simulink library "ITKLib"  (R2022b)
settings: Solver=FixedStepDiscrete  StartTime=0.0  StopTime=10.0  FixedStep=0.01  RelTol=1e-3  EnableMultiTasking=on
values from neighbouring files (symbols this model uses):
  Glb_WhlRollgRd_SC = single(0.36)    [init_Global.m]
undefined symbols (not defined in the file or in its folder): docblock, SlDemoSign, SlDemoSign_Positive_SC, TaskTime_100ms_SC, TaskTime_10ms_SC, VehRefSpd_vMaxRefSpd_C
libraries: simulink x51, $bdroot x45, ITKLib_V14 x1
(part 1 of 10)
settings Model: Creator=MaoChongchong  LastModifiedBy=shuli1
settings SolverCC: AlgebraicLoopSolver=TrustRegion
settings DataIOCC: LimitDataPoints=on  SaveOutput=off  SaveTime=off  ReturnWorkspaceOutputs=off
settings OptimizationCC: DefaultParameterBehavior=Inlined  LifeSpan=1  EfficientTunableParamExpr=on
settings DebuggingCC: UnconnectedInputMsg=warning  UnconnectedOutputMsg=warning  UnconnectedLineMsg=warning  AllowSymbolicDim=off  SFUnexpectedBacktrackingDiag=warning  SFNoUnconditionalDefaultTransitionDiag=warning  SFExecutionAtInitializationDiag=none  SFMachineParentedDataDiag=warning  ArithmeticOperatorsInVariantConditions=warning
settings ModelReferenceCC: EnableRefExpFcnMdlSchedulingChecks=on  PropagateSignalLabelsOutOfModel=off
settings SFSimCC: SimUseLocalCustomCode=off  MATLABDynamicMemAlloc=off  CustomCodeUndefinedFunction=UseInterfaceOnly
settings RTWCC: Description=Embedded Coder  SystemTargetFile=ert.tlc  TemplateMakefile=ert_default_tmf  RTWUseLocalCustomCode=off  DLArmComputeVersion=19.05
settings CodeAppCC: IgnoreCustomStorageClasses=off  StateflowObjectComments=on
settings ERTTargetCC: MultiwordLength=2048  GenerateSampleERTMain=on  InlinedParameterPlacement=NonHierarchical  ERTCustomFileTemplate=example_file_process.tlc  ConvertIfToSwitch=off  SuppressUnreachableDefaultCases=off
settings ConfigComp: CovMetricSettings=dw  CovSaveCumulativeToWorkspaceVar=on  CovSaveSingleToWorkspaceVar=on  CovExternalEMLEnable=off

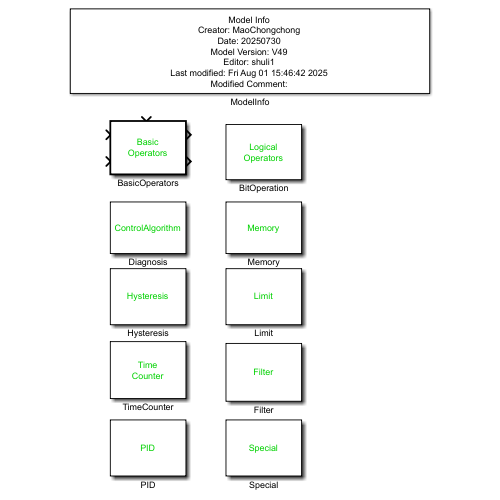
[thumbnail: Simulink's stored preview of the top-level diagram]
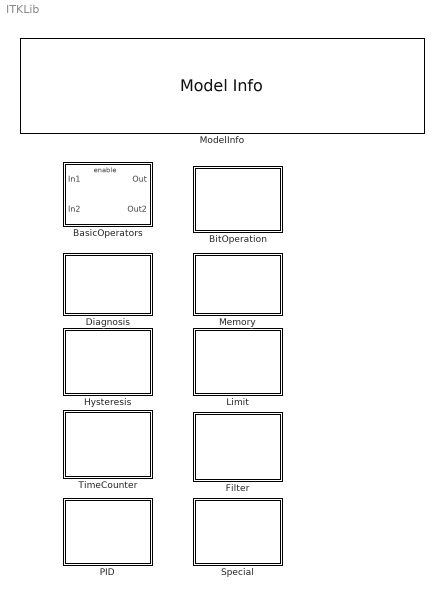
== system ITKLib ==
  BasicOperators : Subsystem
      mask Display:
      | color('green')
      | fprintf('Basic\nOperators')
  BitOperation : Subsystem
      mask Display:
      | color('green')
      | fprintf('Logical\nOperators')
  Diagnosis : Subsystem
      mask Display:
      | color('green')
      | fprintf('ControlAlgorithm')
  Filter : Subsystem
      mask Display:
      | color('green')
      | fprintf('Filter')
  Hysteresis : Subsystem
      mask Display:
      | color('green')
      | fprintf('Hysteresis')
  Limit : Subsystem
      mask Display:
      | color('green')
      | fprintf('Limit')
  Memory : Subsystem
      mask Display:
      | color('green')
      | fprintf('Memory')
  ModelInfo : simulink/Model-Wide Utilities/Model Info  Frame=on  DisplayStringWithTags=|  HorizontalTextAlignment=Center  LeftAlignmentValue=0.5
      | Model Info
      | Creator: MaoChongchong
      | Date: 20250730
      | Model Version: V49
      | Editor: %<LastModifiedBy>
      | Last modified: %<ModifiedDate>
      | Modified Comment:
  PID : Subsystem
      mask Display:
      | color('green')
      | fprintf('PID')
  Special : Subsystem  Description=Refer Detailed Function Description for detailed information.
      mask Display:
      | color('green')
      | fprintf('Special')
  TimeCounter : Subsystem
      mask Display:
      | color('green')
      | fprintf('Time\nCounter')

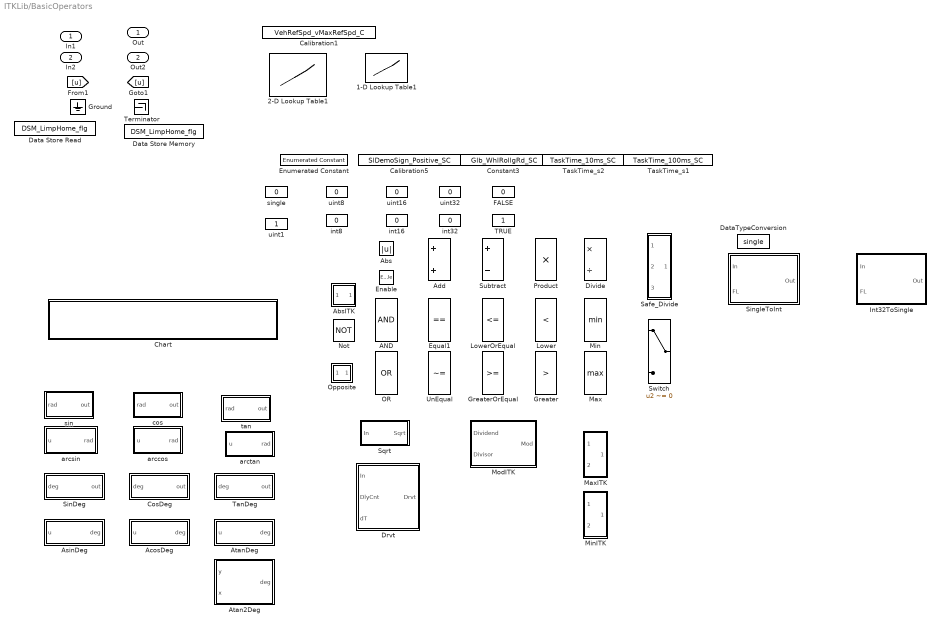
== system ITKLib/BasicOperators ==
  In1 : Inport
  In2 : Inport  Port=2
  Enable : EnablePort
  1-D Lookup Table1 : Lookup_n-D  NumberOfTableDimensions=1  BreakpointsForDimension1=[-5:5]  BreakpointsForDimension1DataTypeStr=Inherit: Inherit from 'Breakpoint data'  Table=tanh([-5:5])  TableDataTypeStr=Inherit: Inherit from 'Table data'  ExtrapMethod=Clip  UseLastTableValue=on  InternalRulePriority=Speed  OutDataTypeStr=Inherit: Inherit from 'Table data'  RndMeth=Simplest
      settings: AttributesFormatString=|
      | input = %<BreakpointsForDimension1>
      | output = %<Table>
      | extrapolation-use end values: %<UseLastTableValue>
  2-D Lookup Table1 : Lookup_n-D  BreakpointsForDimension1=[1:3]  BreakpointsForDimension2=[1:3]  BreakpointsForDimension1DataTypeStr=Inherit: Inherit from 'Breakpoint data'  BreakpointsForDimension2DataTypeStr=Inherit: Inherit from 'Breakpoint data'  TableDataTypeStr=Inherit: Inherit from 'Table data'  ExtrapMethod=Clip  UseLastTableValue=on  InternalRulePriority=Speed  OutDataTypeStr=Inherit: Inherit from 'Table data'  RndMeth=Simplest  InputSameDT=off
      settings: InputPortMap=u0,u1
      settings: AttributesFormatString=|
      | row = %<BreakpointsForDimension1>
      | column = %<BreakpointsForDimension2>
      | output = %<Table>
      | extrapolation-use end values: %<UseLastTableValue>
  AND : Logic  OutDataTypeStr=boolean
  Abs : Abs  SaturateOnIntegerOverflow=off  OutDataTypeStr=Inherit: Inherit via internal rule
  AbsITK : Subsystem  mask(AbsITK){}
      mask help: This block returns the absolute value of input
      mask Display:
      | color('blue')
      | disp('\fontsize{12}Abs', 'texmode', 'on')
      | color('green');
      | text(1,0,'ITK','horizontalAlignment','right','verticalAlignment','bottom');
  AcosDeg : Subsystem  mask(Acos){}
      mask help:
      | This block returns the sin of an angle
      | Result = acos(value)
      | Input:
      |             u: input value, the maximum value is 1, the minimum value is -1;
      | Output:
      |             out: angle, unit: deg, the maximum value is 180 deg, the minimum value is 0 deg;
      mask Display:
      | color('blue')
      | disp('\fontsize{10}acos', 'texmode', 'on')
      | color('green');
      | text(1,0,'ITK','horizontalAlignment','right','verticalAlignment','bottom');
  Add : Sum  InputSameDT=on  SaturateOnIntegerOverflow=on
  AsinDeg : Subsystem  mask(AsinDeg){}
      mask help:
      | This block returns the sin of an angle
      | Result = asin(value)
      | Input:
      |             u: input value, the maximum value is 1, the minimum value is -1;
      | Output:
      |             out: angle, unit: deg, the maximum value is 90 deg, the minimum value is -90 deg;
      mask Display:
      | color('blue')
      | disp('\fontsize{10}asin', 'texmode', 'on')
      | color('green');
      | text(1,0,'ITK','horizontalAlignment','right','verticalAlignment','bottom');
  Atan2Deg : Subsystem  mask(Atan2Deg){}
      mask help:
      | This block returns the sin of an angle
      | Result = atan2(value)
      | Input:
      |             u: input value, the maximum value is 5729, the minimum value is -5729;
      | Output:
      |             out: angle, unit: deg, the maximum value is 179.99 deg, the minimum value is -179.99 deg, does not include from -89.99 deg to -90 deg and from 89.99 deg to 90 deg;
      mask Display:
      | color('blue')
      | disp('\fontsize{10}atan2', 'texmode', 'on')
      | color('green');
      | text(1,0,'ITK','horizontalAlignment','right','verticalAlignment','bottom');
  AtanDeg : Subsystem  mask(Atan){}
      mask help:
      | This block returns the sin of an angle
      | Result = atan(value)
      | Input:
      |             u: input value, the maximum value is 5729, the minimum value is -5729;
      | Output:
      |             out: angle, unit: deg, the maximum value is 89.99 deg, the minimum value is -89.99 deg;
      mask Display:
      | color('blue')
      | disp('\fontsize{10}atan', 'texmode', 'on')
      | color('green');
      | text(1,0,'ITK','horizontalAlignment','right','verticalAlignment','bottom');
  Calibration1 : Constant  Description=[300]  Value=VehRefSpd_vMaxRefSpd_C  SampleTime=-1
      settings: AttributesFormatString=%<Description>
  Calibration5 : Constant  Description=[0]  Value=SlDemoSign_Positive_SC  SampleTime=-1
      settings: AttributesFormatString=%<Description>
  Chart : Stateflow chart  TreatAsAtomicUnit=on
  Constant3 : Constant  Description=[0.36]  Value=Glb_WhlRollgRd_SC  SampleTime=-1
      settings: AttributesFormatString=%<Description>
  CosDeg : Subsystem  mask(CosDeg){}
      mask help:
      | This block returns the sin of an angle
      | Result = cos(value)
      | Input:
      |             deg: input angle, unit: deg, the minimum value is -inf, the maximum value is inf;
      | Output:
      | out: the minimum value is -1, the maximum value is 1;
      mask Display:
      | color('blue')
      | disp('\fontsize{10}cos(deg)', 'texmode', 'on')
      | color('green');
      | text(1,0,'ITK','horizontalAlignment','right','verticalAlignment','bottom');
  Data Store Memory : DataStoreMemory  DataStoreName=DSM_LimpHome_flg  ReadBeforeWriteMsg=warning  WriteAfterWriteMsg=warning  WriteAfterReadMsg=warning  ShowAdditionalParam=off  OutDataTypeStr=boolean
  Data Store Read : DataStoreRead  DataStoreName=DSM_LimpHome_flg  DataStoreElements=DSM_LimpHome_flg  IndexOptions=Index vector (dialog)  Indices=1  OutputSizes=1
  DataTypeConversion : DataTypeConversion  OutDataTypeStr=single  RndMeth=Nearest  SaturateOnIntegerOverflow=off
  Divide : Product  Inputs=*/  InputSameDT=on  SaturateOnIntegerOverflow=on
  Drvt : Subsystem  mask(Drvt){}
      mask help:
      | This block returns the derivativee value of input signal.
      |
      | Input signals:
      |             In: input signal, single data type;
      |             DlyCnt: delay counter value, uint data type;
      |             dT: sample time, single data type, unit is s;
      | Output:
      |             Drvt: derivativee value of In, single data type;
      settings: MinAlgLoopOccurrences=on
      mask Display:
      | color('blue')
      | % disp('\fontsize{10}Drvt', 'texmode', 'on')
      | color('green');
      | % image('SqrtImage.jpg', 'center');
      | image('DrvtImage.jpg', [0.36, 0.3, 0.42, 0.5]);
      | text(1,0,'ITK','horizontalAlignment','right','verticalAlignment','bottom');
  Enumerated Constant : simulink/Sources/Enumerated Constant  OutDataTypeStr=Enum: SlDemoSign  Value=SlDemoSign.Positive  SampleTime=-1
  Equal1 : RelationalOperator  Operator===  OutDataTypeStr=boolean
  FALSE : Constant  Description=FALSE  Value=0  OutDataTypeStr=boolean  SampleTime=-1
      settings: AttributesFormatString=%<Description>
  Greater : RelationalOperator  Operator=>  OutDataTypeStr=boolean
  GreaterOrEqual : RelationalOperator  OutDataTypeStr=boolean
  Ground : Ground
  Int32ToSingle : Subsystem  mask(Int32ToSingle){}
      mask help:
      | Convert int32 number to single number using binary point scaling with specified fraction length (FL).
      | Equivalent to fixdt(1,32,FL) from Fix-point Designer toolbox
      | Input:
      |             In: input signal, int32 data type;
      |             FL: specified fraction length, single data type, ＞0；
      | Output:
      |             Out: output signal, single data type;
      mask Display:
      | color('blue')
      | disp('\fontsize{10}Int32ToSingle', 'texmode', 'on')
      | color('green');
      | % image('SqrtImage.jpg', 'center');
      | % image('SqrtImage.jpg', [0.25, 0.2, 0.4, 0.6]);
      | text(1,0,'ITK','horizontalAlignment','right','verticalAlignment','bottom');
  Lower : RelationalOperator  Operator=<  OutDataTypeStr=boolean
  LowerOrEqual : RelationalOperator  Operator=<=  OutDataTypeStr=boolean
  Max : MinMax  Function=max  Inputs=2  InputSameDT=on  SaturateOnIntegerOverflow=on
  MaxITK : Subsystem  mask(MaxITK){}
      mask help: This block returns the maximal value of input
      mask Display:
      | color('blue')
      | disp('\fontsize{12}Max', 'texmode', 'on')
      | color('green');
      | text(1,0,'ITK','horizontalAlignment','right','verticalAlignment','bottom');
  Min : MinMax  Inputs=2  InputSameDT=on  SaturateOnIntegerOverflow=on
  MinITK : Subsystem  mask(MinITK){}
      mask help: This block returns the minimum value of input
      mask Display:
      | color('blue')
      | disp('\fontsize{12}Min', 'texmode', 'on')
      | color('green');
      | text(1,0,'ITK','horizontalAlignment','right','verticalAlignment','bottom');
  ModITK : Subsystem  mask(ModITK){}
      mask help:
      | This block returns the mod of Dividend/Divisor.
      | Mod = Dividend - fix(Dividend/Divisor)*Divisor
      | Input:
      |             Dividend: ＞0
      |             Divisor: ;＞0
      | Output:
      |             Mod: ;
      mask Display:
      | color('blue')
      | disp('\fontsize{12}Mod', 'texmode', 'on')
      | color('green');
      | % image('SqrtImage.jpg', 'center');
      | % image('SqrtImage.jpg', [0.25, 0.2, 0.4, 0.6]);
      | text(1,0,'ITK','horizontalAlignment','right','verticalAlignment','bottom');
  Not : Logic  Operator=NOT  AllPortsSameDT=off  OutDataTypeStr=boolean
  OR : Logic  Operator=OR  OutDataTypeStr=boolean
  Opposite : Subsystem  RTWFcnName=Minus  RTWFileName=MCC_Mdl_Lib  mask(Opposite){}
      mask help:
      | output = - input;
      | Simulink Custom Model Library, created by MCC.
      settings: RTWFcnNameOpts=User specified  RTWFileNameOpts=User specified
      mask Display:
      | color('blue')
      | fprintf('-ln  ')
      | color('green');
      | % text(1,0,'SEN','horizontalAlignment','right','verticalAlignment','bottom');
  Product : Product  InputSameDT=on  SaturateOnIntegerOverflow=on
  Safe_Divide : Subsystem  RTWFcnName=Safe_Divide  RTWFileName=BoschITK_Mdl_Lib  mask(Safe_Divide){}
      mask help:
      | Safe Divide, prevents division by zero.
      |
      | if abs(denominator) > abs(eps) then
      |     output = numerator / denominator
      | elseif  denominator ≥ 0
      |     output = numerator / abs(eps)
      | else
      |     output = numerator / (-abs(eps))
      |
      |
      | Warning!
      | Use this block only when there is a risk for division by zero.
      |
      | Simulink Custom Model Library, created by MCC.
      settings: RTWFcnNameOpts=User specified  RTWFileNameOpts=User specified
      mask Display:
      | port_label('input', 1, 'x')
      | port_label('input', 2, '÷')
      | port_label('input', 3, 'eps')
  SinDeg : Subsystem  mask(SinDeg){}
      mask help:
      | This block returns the sin of an angle
      | Result = sin(value)
      | Input:
      |             deg: input angle, unit: deg, the minimum value is -inf, the maximum value is inf;
      | Output:
      | out: the minimum value is -1, the maximum value is 1;
      mask Display:
      | color('blue')
      | disp('\fontsize{10}sin(deg)', 'texmode', 'on')
      | color('green');
      | text(1,0,'ITK','horizontalAlignment','right','verticalAlignment','bottom');
  SingleToInt : Subsystem  mask(SingleToInt32){}
      mask help:
      | Convert single number to int32 number using binary point scaling with specified fraction length (FL).
      | Equivalent to fixdt(1,32,FL) from Fix-point Designer toolbox.
      | Input:
      |             In: input signal, single data type;
      |             FL: specified fraction length, single data type, ＞0；
      | Output:
      |             Out: output signal, int32 data type;
      mask Display:
      | color('blue')
      | disp('\fontsize{10}SingleToInt32', 'texmode', 'on')
      | color('green');
      | % image('SqrtImage.jpg', 'center');
      | % image('SqrtImage.jpg', [0.25, 0.2, 0.4, 0.6]);
      | text(1,0,'ITK','horizontalAlignment','right','verticalAlignment','bottom');
  Sqrt : Subsystem  mask(Sqrt){}
      mask help:
      | This block returns the square root value of input signal, according to Newton's iterative method.
      | Sqrt = sqrt(In)
      | Input:
      |             In: input signal, ≥0;
      | Output:
      |             Sqrt: the square root of In, ≥0;
      |  If 0≤ In ≤ 1e13, the output signal Sqrt is right, it has no error;
      |  If  In ＞ 1e13, the output signal Sqrt is not right, it will generate big error;
      mask Display:
      | color('blue')
      | disp('\fontsize{10}Sqrt', 'texmode', 'on')
      | color('green');
      | % image('SqrtImage.jpg', 'center');
      | image('SqrtImage.jpg', [0.25, 0.2, 0.4, 0.6]);
      | text(1,0,'ITK','horizontalAlignment','right','verticalAlignment','bottom');
  Subtract : Sum  Inputs=+-  InputSameDT=on  SaturateOnIntegerOverflow=on
  Switch : Switch  Criteria=u2 ~= 0  SaturateOnIntegerOverflow=off  InputSameDT=off
      settings: AttributesFormatString=Criteria : %<Criteria>
  TRUE : Constant  Description=TRUE  OutDataTypeStr=boolean  SampleTime=-1
      settings: AttributesFormatString=%<Description>
  TanDeg : Subsystem  mask(TanDeg){}
      mask help:
      | This block returns the sin of an angle
      | Result = tan(value)
      | Input:
      |             deg: input angle, unit: deg, the minimum value is -inf, the maximum value is inf, does not include integer multiple angle values of 90 degrees;
      | Output:
      | out: the minimum value is -573, the maximum value is 573;
      mask Display:
      | color('blue')
      | disp('\fontsize{10}tan(deg)', 'texmode', 'on')
      | color('green');
      | text(1,0,'ITK','horizontalAlignment','right','verticalAlignment','bottom');
  TaskTime_s1 : Constant  Description=[0.1]  Value=TaskTime_100ms_SC  SampleTime=-1
      settings: AttributesFormatString=%<Description>
  TaskTime_s2 : Constant  Description=[0.01]  Value=TaskTime_10ms_SC  SampleTime=-1
      settings: AttributesFormatString=%<Description>
  Terminator : Terminator
  UnEqual : RelationalOperator  Operator=~=  OutDataTypeStr=boolean
  arccos : Subsystem  mask(arccos){}
      mask help:
      | This block returns the arccos of an angle
      | Result = arccos(value)
      mask Display:
      | color('blue')
      | disp('\fontsize{10}arccos', 'texmode', 'on')
      | color('green');
      | text(1,0,'ITK','horizontalAlignment','right','verticalAlignment','bottom');
  arcsin : Subsystem  mask(arcsin){}
      mask help:
      | Returns the inverse sine of an angle, in the range of -pi/2 through pi/2.
      | If the argument is zero, then the result is a zero
      | Result = arcsin(value)
      mask Display:
      | color('blue')
      | disp('\fontsize{10}arcsin', 'texmode', 'on')
      | color('green');
      | text(1,0,'ITK','horizontalAlignment','right','verticalAlignment','bottom');
  arctan : Subsystem  mask(arctan){}
      mask help:
      | This block returns the arctan of an angle
      | Result = arctan(value)
      mask Display:
      | color('blue')
      | disp('\fontsize{10}arctan', 'texmode', 'on')
      | color('green');
      | text(1,0,'ITK','horizontalAlignment','right','verticalAlignment','bottom');
  cos : Subsystem  mask(cos){}
      mask help:
      | This block returns the cos of an angle
      | Result = cos(value)
      mask Display:
      | color('blue')
      | disp('\fontsize{10}cos', 'texmode', 'on')
      | color('green');
      | text(1,0,'ITK','horizontalAlignment','right','verticalAlignment','bottom');
  int16 : Constant  Value=0  OutDataTypeStr=int16  SampleTime=-1
      settings: AttributesFormatString=%<OutDataTypeStr>
  int32 : Constant  Value=0  OutDataTypeStr=int32  SampleTime=-1
      settings: AttributesFormatString=%<OutDataTypeStr>
  int8 : Constant  Value=0  OutDataTypeStr=int8  SampleTime=-1
      settings: AttributesFormatString=%<OutDataTypeStr>
  sin : Subsystem  mask(Sin){}
      mask help:
      | This block returns the sin of an angle
      | Result = sin(value)
      mask Display:
      | color('blue')
      | disp('\fontsize{10}sin', 'texmode', 'on')
      | color('green');
      | text(1,0,'ITK','horizontalAlignment','right','verticalAlignment','bottom');
  single : Constant  Value=0  OutDataTypeStr=single  SampleTime=-1
      settings: AttributesFormatString=%<OutDataTypeStr>
  tan : Subsystem  mask(tan){}
      mask help:
      | This block returns the tan of an angle
      | Result = tan(value)
      mask Display:
      | color('blue')
      | disp('\fontsize{10}tan', 'texmode', 'on')
      | color('green');
      | text(1,0,'ITK','horizontalAlignment','right','verticalAlignment','bottom');
  uint1 : Constant  Description=Connect  OutDataTypeStr=uint8  SampleTime=-1
      settings: AttributesFormatString=|
      | %<OutDataTypeStr>
      | %<Description>
  uint16 : Constant  Value=0  OutDataTypeStr=uint16  SampleTime=-1
      settings: AttributesFormatString=%<OutDataTypeStr>
  uint32 : Constant  Value=0  OutDataTypeStr=uint32  SampleTime=-1
      settings: AttributesFormatString=%<OutDataTypeStr>
  uint8 : Constant  Value=0  OutDataTypeStr=uint8  SampleTime=-1
      settings: AttributesFormatString=%<OutDataTypeStr>
  Out : Outport  VectorParamsAs1DForOutWhenUnconnected=off
  Out2 : Outport  Port=2  VectorParamsAs1DForOutWhenUnconnected=off

== system ITKLib/BitOperation ==
  GetBitU16 : Subsystem  mask(GetBit_U16){}
      mask help:
      | Pos: Designated bits position of the input signal which want to get, uint8 data type, the minimum value is 0, the maximum value is 15.
      | In: Input signal, uint16 data type
      | If the bit position exceed the range of input quantity, output is false.
      | Simulink Custom Model Library, created by MCC.
      mask Display:
      | color('blue')
      | disp('\fontsize{12}GetBitU16', 'texmode', 'on')
      | color('green');
      | text(1,0,'ITK','horizontalAlignment','right','verticalAlignment','bottom');
  GetBitU32 : Subsystem  mask(GetBit_U32){}
      mask help:
      | Pos: Designated bits position of the input signal which want to get, the minimum value is 0, the maximum value is 31.
      | In: Input signal, uint32 data type
      | If the bit position exceed the range of input quantity, output is false.
      | Simulink Custom Model Library, created by MCC.
      mask Display:
      | color('blue')
      | disp('\fontsize{12}GetBitU32', 'texmode', 'on')
      | color('green');
      | text(1,0,'ITK','horizontalAlignment','right','verticalAlignment','bottom');
  GetBitU8 : Subsystem  RTWFcnName=GetBitU8  RTWFileName=ITKC_Mdl_Lib  mask(GetBit_U8){}
      mask help:
      | Pos: Designated bits position of the input signal which want to get, uint8 data type, the minimum value is 0, the maximum value is 7.
      | In: Input signal, uint8 data type
      | If the bit position exceed the range of input quantity, output is false.
      | Simulink Custom Model Library, created by MCC.
      settings: RTWFcnNameOpts=User specified  RTWFileNameOpts=User specified
      mask Display:
      | color('blue')
      | disp('\fontsize{12}GetBitU8', 'texmode', 'on')
      | color('green');
      | text(1,0,'ITK','horizontalAlignment','right','verticalAlignment','bottom');
  MaskAnd : Subsystem  mask(BitMask){}
      mask help:
      | Comapre the bit value of 'In' and 'Mask'.
      | Summary the bit which are se to 1 in 'Mask' and if the corresponding bit are set to 1 in 'In' also, the 'Out' is 1.
      | Otherwise, the 'Out' is 0.
      | If Mask = 0, the Out is 0.
      mask Display:
      | color('blue')
      | disp('\fontsize{12}Mask And', 'texmode', 'on')
      | color('green');
      | text(1,0,'ITK','horizontalAlignment','right','verticalAlignment','bottom');
  MaskOr : Subsystem  RTWFcnName=MaskOr  RTWFileName=MCC_Mdl_Lib  mask(BitMaskOr){}
      mask help:
      | Comapre the bit value of 'In' and 'Mask'.
      | Summary the bit which are set to 1 in 'Mask' and if the corresponding bit are set to 1 in 'In' also, the 'Out' is 1.
      | Otherwise, the 'Out' is 0.
      | If Mask = 0, the Out is 0.
      settings: MinAlgLoopOccurrences=on  RTWFcnNameOpts=User specified  RTWFileNameOpts=User specified
      mask Display:
      | color('blue')
      | disp('\fontsize{12}Mask Or', 'texmode', 'on')
      | color('green');
      | text(1,0,'ITK','horizontalAlignment','right','verticalAlignment','bottom');
  Merge16bit2out : Subsystem  RTWFcnName=Merge16bit2out  RTWFileName=MCC_Mdl_Lib  mask(16bit2out){}
      mask help:
      | 8bit2out
      | Simulink Custom Model Library, created by MCC.
      settings: AttributesFormatString=Merge16bit2out  RTWFcnNameOpts=User specified  RTWFileNameOpts=User specified
      mask Display:
      | color('green');
      | text(1,0,'ITK','horizontalAlignment','right','verticalAlignment','bottom');
  Merge20bit2out : Subsystem  mask(Merge20bit2out){}
      mask help: Merge 20 bits into 1 LWord
      mask Display:
      | color('blue')
      | disp('\fontsize{12}Merge Bit', 'texmode', 'on')
      | color('green');
      | text(1,0,'ITK','horizontalAlignment','right','verticalAlignment','bottom');
  Merge2bit2out : Subsystem  mask(Merge2bit2out){}
      mask help: Merge 2 bits into 1 LWord
      mask Display:
      | color('blue')
      | disp('\fontsize{12}Merge Bit', 'texmode', 'on')
      | color('green');
      | text(1,0,'ITK','horizontalAlignment','right','verticalAlignment','bottom');
  Merge32bit2out : Subsystem  RTWFcnName=Merge16bit2out  RTWFileName=MCC_Mdl_Lib  mask(32bit2out){}
      mask help:
      | 32bit2out
      | Simulink Custom Model Library, created by MCC.
      settings: AttributesFormatString=Merge32bit2out  RTWFcnNameOpts=User specified  RTWFileNameOpts=User specified
      mask Display:
      | color('green');
      | text(1,0,'ITK','horizontalAlignment','right','verticalAlignment','bottom');
  Merge3bit2out : Subsystem  mask(Merge3bit2out){}
      mask help: Merge3 bits into 1 LWord
      mask Display:
      | color('blue')
      | disp('\fontsize{12}Merge Bit', 'texmode', 'on')
      | color('green');
      | text(1,0,'ITK','horizontalAlignment','right','verticalAlignment','bottom');
  Merge4bit2out : Subsystem  mask(Merge4bit2out){}
      mask help: Merge 4 bits into 1 LWord
      mask Display:
      | color('blue')
      | disp('\fontsize{12}Merge Bit', 'texmode', 'on')
      | color('green');
      | text(1,0,'ITK','horizontalAlignment','right','verticalAlignment','bottom');
  Merge5bit2out : Subsystem  mask(Merge5bit2out){}
      mask help: Merge 5 bits into 1 LWord
      mask Display:
      | color('blue')
      | disp('\fontsize{12}Merge Bit', 'texmode', 'on')
      | color('green');
      | text(1,0,'ITK','horizontalAlignment','right','verticalAlignment','bottom');
  Merge6bit2out : Subsystem  mask(Merge6bit2out){}
      mask help: Merge 6 bits into 1 LWord
      mask Display:
      | color('blue')
      | disp('\fontsize{12}Merge Bit', 'texmode', 'on')
      | color('green');
      | text(1,0,'ITK','horizontalAlignment','right','verticalAlignment','bottom');
  Merge7bit2out : Subsystem  mask(Merge7bit2out){}
      mask help: Merge 7 bits into 1 LWord
      mask Display:
      | color('blue')
      | disp('\fontsize{12}Merge Bit', 'texmode', 'on')
      | color('green');
      | text(1,0,'ITK','horizontalAlignment','right','verticalAlignment','bottom');
  Merge8bit2out : Subsystem  RTWFcnName=Merge8bit2out  RTWFileName=MCC_Mdl_Lib  mask(8bit2out){}
      mask help:
      | 8bit2out
      | Simulink Custom Model Library, created by MCC.
      settings: AttributesFormatString=Merge8bit2out  MinAlgLoopOccurrences=on  RTWFcnNameOpts=User specified
      mask Display:
      | color('green');
      | text(1,0,'ITK','horizontalAlignment','right','verticalAlignment','bottom');
  Subsystem : Subsystem  mask(PutBit_U8){}
      mask help:
      | Pos: Designated bits position of the input signal to be put
      | BitVal: the modified bit value
      | In: Input signal
      | If the bit position exceed the range of input quantity, output the input directly
      mask Display:
      | color('blue')
      | disp('\fontsize{12}PutBit', 'texmode', 'on')
      | color('green');
      | text(1,0,'ITK','horizontalAlignment','right','verticalAlignment','bottom');
  Subsystem1 : Subsystem  mask(GetBit_U8){}
      mask help:
      | Pos: Designated bits position of the input signal which want to get
      | In: Input signal
      | If the bit position exceed the range of input quantity, output the input directly
      mask Display:
      | color('blue')
      | disp('\fontsize{12}GetBit', 'texmode', 'on')
      | color('green');
      | text(1,0,'ITK','horizontalAlignment','right','verticalAlignment','bottom');
  Subsystem2 : Subsystem  mask(SetBit_U8){}
      mask help:
      | Pos: Designated bits position of the input signal to be set to 1
      | In: Input signal
      | If the bit position exceed the range of input quantity, output the input directly
      mask Display:
      | color('blue')
      | disp('\fontsize{12}SetBit', 'texmode', 'on')
      | color('green');
      | text(1,0,'ITK','horizontalAlignment','right','verticalAlignment','bottom');

== system ITKLib/Diagnosis ==
  CheckSum_SGMW : Subsystem  RTWFcnName=CheckSum_SGMW  RTWFileName=JaevRI_Mdl_Lib  mask(CheckSumErr_SGMW){}
      mask help:
      | This block is used to calculate CheckSum value and error flag :
      | Input: Byte0 ~Byte6, single type, maximum value is 255, minimum value is 0;
      |          CheckSumVal, single type, the compared value from CAN communication;
      | Output: CheckSumCal, single type, the calculated checksum value;
      |             CheckSumErr, boolean type, CheckSumErr is true when CheckSumCal is not equal to CheckSumVal, CheckSumErr is false when CheckSumCal is equal to CheckSumVal;
      | CheckSum Calculation rule：
      |        Byte0 + Byte1 +Byte2 +Byte3 +Byte4 +Byte5 + Byte6，hexadecimal addition without carry;
      |       For example, Byte0 is 8C, Byte1 is 9D, Byte2 is 00, Byte3 is 00, Byte4 is 00, Byte5 is 00, Byte6 is 00,
      |       CheckSumCal = Byte0 + Byte1 +Byte2 +Byte3 +Byte4 +Byte5 + Byte6 = 8C + 9D + 00 + 00 + 00 + 00 + 00 = 19;
      |
      | Simulink Custom Model Library, created by MCC.
      settings: AttributesFormatString=CheckSum  RTWFcnNameOpts=User specified  RTWFileNameOpts=User specified
      mask Display:
      | color('blue')
      | % dpoly(1,[1 0],'z')
      | disp('\fontsize{12}CheckSum', 'texmode', 'on')
      | color('green');
      | text(1,0,'ITK','horizontalAlignment','right','verticalAlignment','bottom');
      | %text(1,0,'SEN','horizontalAlignment','right','verticalAlignment','bottom');
  Crc16Gen : MATLAB Function
      settings: MinAlgLoopOccurrences=on
  Crc8Gen : MATLAB Function
      settings: MinAlgLoopOccurrences=on
  Debounce_OBD : Subsystem  RTWFcnName=Debounce_OBD  RTWFileName=JaevRI_Mdl_Lib  mask(Debounce_OBD_FCN_SL){}
      mask help:
      | ITK Library for Function Development
      |
      | ISO 14229 D.5  DTC-FaultDetectionCounter operation definition
      | Inputs:
      | bErr     Error signal(s)  (i.e. vector of continuous test runs)
      | FailThd      counter a value between 0 and 32767  (for each bErr signal)
      | RecThd  counter a value between 0 and -32768 (for each bErr signal)
      | IncrFail     increment Fault counter (>0) max 255 in timer ticks for each signal
      | DecrRec      decrement Recovery counter (<0) min -128 in timer ticks for each signal
      | bEna    bErr is 0 when bEna=0, detecting whether bErr is 1 when bEna=1
      | bRst     reset flag of bErr(bErr is 0 when bRst=1)
      | So Counters are in numbers of timer ticks of TaskTime_s(=0.01s);
      | E.g. if Increment counter is 5 and decrement counter -3,
      | then maximum fail times are: 32767*0.01/5 = 65.534 sec,
      | maximum recovery times are: -32768*0.01/3 = 109.2267 sec;
      | E.g. if FailThd is 20, RecThd is -4, Increment counter is 5 and decrement counter -3 when bEna is 1and bRst is 0,
      | then fail times are: 20*0.01/5 = 0.04 sec, recovery times are: (-4-20)*0.01/(-3) = 0.08 sec;
      |
      | Outputs :
      | bFailed testFailed  (Bit 0)
      |
      | Notes:
      | * Outputs are held when input bEna is disabled
      | * Due to Int16 instead of Int8 and Incr/Decr 5/-3 by default the above mentioned ISO standard is somewhat changed.
      |
      | Simulink Custom Model Library, created by MCC.
      settings: RTWFcnNameOpts=User specified  RTWFileNameOpts=User specified
      mask Display:
      | % color('black');
      | % plot([0.2,0.2],[0.1,0.9]);
      | % plot([0.205,0.205],[0.1,0.9]);
      | % plot([0.2,0.8],[0.8,0.8]);
      | % plot([0.2,0.8],[0.65,0.65]);
      | % plot([0.2,0.8],[0.45,0.45]);
      | % plot([0.2,0.8],[0.25,0.25]);
      | % plot([0.2,0.8],[0.1,0.1]);
      | port_label('input',1,'bErr');
      | port_label('input',2,'bRst');
      | port_label('input',3,'bEna');
      | port_label('input',4,'FailThd');
      | port_label('input',5,'RecThd');
      | port_label('input',6,'IncrFail');
      | port_label('input',7,'DecrRec');
      | port_label('output',1,'bFailed');
      | color('blue');
      | disp('\fontsize{12}Debounce', 'texmode', 'on')
      | color('green');
      | text(1,0,'ITK','horizontalAlignment','right','verticalAlignment','bottom');
      | % color('cyan');
      | % plot([0.3,0.3],[0.1,0.9]);
      | % plot([0.4,0.4],[0.1,0.9]);
      | % plot([0.5,0.5],[0.1,0.9]);
      | % plot([0.6,0.6],[0.1,0.9]);
      | % plot([0.7,0.7],[0.1,0.9]);
      | % plot([0.8,0.8],[0.1,0.9]);
      | % color('orange');
      | % plot([0.2,0.3,0.3,0.6,0.6,0.8],[0.85,0.85,0.8,0.8,0.85,0.85]);
      | % plot([0.2,0.5,0.5,0.6,0.6,0.8],[0.7,0.7,0.65,0.65,0.7,0.7]);
      | % color('blue');
      | % plot([0.2,0.3,0.4,0.5,0.5,0.6,0.7,0.8],[0.45,0.55,0.35,0.35,0.45,0.45,0.6,0.6]);
      | % color('red');
      | % plot([0.2,0.7,0.7,0.8],[0.25,0.25,0.3,0.3]);
      | % color('green');
      | % plot([0.2,0.4,0.4,0.5,0.5,0.8],[0.1,0.1,0.15,0.15,0.1,0.1]);
  FltCollctn : Subsystem  RTWFcnName=RCChk_0_15  RTWFileName=JaevRI_Mdl_Lib  mask(FltCollctn){}
      mask help:
      | This block is used to collect fault based on falut falg and fault number.
      | Input:
      |           FltFlg, fault flag, boolean data type;
      |           FltNr, fault number, uint8 data type;
      | Output:
      |           BatProt_stFltCodAry, [1 16 ] array uint16 data, this signal summarizes the fault flag bits into uint16 data, different bits indicate different faults, corresponding to whether the FltFlg  is 1;
      |           BatProt_stFltAry, [1 255] array uint8 data, if the value of corresponding bit is 16, the FltFlg of corresponding bit is true.
      |
      | Simulink Custom Model Library, created by MCC.
      settings: RTWFcnNameOpts=User specified  RTWFileNameOpts=User specified
      mask Display:
      | color('blue')
      | % dpoly(1,[1 0],'z')
      | disp('\fontsize{12}FltCollctn', 'texmode', 'on')
      | color('green');
      | text(1,0,'ITK','horizontalAlignment','right','verticalAlignment','bottom');
      | %text(1,0,'SEN','horizontalAlignment','right','verticalAlignment','bottom');
  FltLatchCollctn : Subsystem  AncestorBlock=ITKLib_V271/Diagnosis/FltLatchCollctn  RTWFcnName=RCChk_0_15  RTWFileName=JaevRI_Mdl_Lib  mask(FltCollctn){}
      mask help:
      | This block is used to collect fault based on falut falg and fault number.
      | Input:
      |           FltFlg, fault flag, boolean data type;
      |           FltNr, fault number, uint8 data type;
      |           SentCod, Sent fault number, uint8 data type, Dimension[1 4];
      | Output:
      |           BatProt_stFltCodAry, [1 16 ] array uint16 data, this signal summarizes the fault flag bits into uint16 data, different bits indicate different faults, corresponding to whether the FltFlg  is 1;
      |           BatProt_stFltAry, [1 255] array uint8 data, if the value of corresponding bit is 16, the FltFlg of corresponding bit is true.
      |           Clear when SentCod appears the value of corresponding bit.
      |
      | Simulink Custom Model Library, created by MCC.
      settings: RTWFcnNameOpts=User specified  RTWFileNameOpts=User specified
      mask Display:
      | color('blue')
      | % dpoly(1,[1 0],'z')
      | disp('\fontsize{12}FltCollctn', 'texmode', 'on')
      | color('green');
      | text(1,0,'ITK','horizontalAlignment','right','verticalAlignment','bottom');
      | %text(1,0,'SEN','horizontalAlignment','right','verticalAlignment','bottom');
  FltMux : Subsystem  RTWFcnName=RCChk_0_15  RTWFileName=JaevRI_Mdl_Lib  mask(FltMux){MaiFltLvl=3, SubFltLvl=1, FltCod=45, ClsIgbtEna=off, TqRdcEna=off, TqRdcFac=100}
      mask prompts: MaiFltLvl "Main Fault Level :"; SubFltLvl "Sub Fault Level :"; FltCod "Fault Code :"; ClsIgbtEna "Close IGBT Enable"; TqRdcEna "Torque Reduce Enable"; TqRdcFac "Torque Reduce Factor :"
      mask help:
      | The module mainly configures fault flag bits for fault classification and fault response actions.
      | Input:
      | FltFlg: fault flag, boolean data type;
      | FltOpenEna: fault open enable flag, boolean data type;
      | Parameters：
      | ClsIgbtEna: Close IGT enable flag, boolean data type;
      | TqRdcEna: Torque reduce enable flag, boolean data type;
      | TqRdcFac: Torque reduce factor, single data type, the maximum value is 100, the minumum value is 0;
      | MaiFltLvl: Main fault level, uint8 data type;
      | SubFltLvl: Sub fault level, uint8 data type;
      | FltCod: Fault code, uint16 data type;
      | Output:
      | FltMax is bus signal, it has the following signals:
      |     MaiFltLvl: The actual main fault level, uint8 data type;
      |     SubFltLvl: The actual sub fault level, uint8 data type;
      |     FltCod: The actual fault code, uint16 data type;
      |     ClsIgbtActv: The actual close IGBT active flag, boolean data type;
      |     TqRdcFac: The actual torque reduce factor, single data type, the maximum value is 1, the minumum value is 0;
      |
      | Simulink Custom Model Library, created by MCC.
      settings: AttributesFormatString=FltMux  RTWFcnNameOpts=User specified  RTWFileNameOpts=User specified
      mask Display:
      | color('blue')
      | gr_opt1 = get_param(gcb,'MaiFltLvl');
      | a = str2num(gr_opt1);
      | gr_opt2 = get_param(gcb,'SubFltLvl');
      | b = str2num(gr_opt2);
      | gr_opt3 = get_param(gcb,'FltCod');
      | c = str2num(gr_opt3);
      | gr_opt4 = get_param(gcb,'ClsIgbtEna');
      | d = str2num(gr_opt4);
      | gr_opt5 = get_param(gcb,'TqRdcEna');
      | e = str2num(gr_opt5);
      | gr_opt6 = get_param(gcb,'TqRdcFac');
      | f = str2num(gr_opt6);
      | fprintf(['主故障等级: %d\n' ...
      |     '子故障等级: %d\n'...
      |     '  故障码       : %d\n'...
      |       '       扭矩限制    : %d%%'],a,b,c,f);
      | color('green');
      | text(1,0,'ITK','horizontalAlignment','right','verticalAlignment','bottom');
  LifeCycleCounter : Subsystem  RTWFcnName=LifeCycleCnt  RTWFileName=MCC_Mdl_Lib  mask(LifeCycCntr){}
      mask help:
      | Increments step by value 1;
      | MaxCnt: the maximum limit count, uint16 data type;
      | LifeCycleCnt range：0 ~ maximum limit，uint16 data type；
      | When counter reaches maximum limit, LifeCycleCnt return to 0;
      |
      | Simulink Custom Model Library, created by MCC.
      settings: MinAlgLoopOccurrences=on  RTWFcnNameOpts=User specified  RTWFileNameOpts=User specified
      mask Display:
      | color('blue')
      | plot(0.05+0.05*[0 1 1 2 2 3 3 4 4 5 5 6 6 7 7 8 8 9 9 10 10 11 11 12 12 13],0.05+0.15*[0 0 1 1 2 2 3 3 4 4 5 5 0 0 1 1 2 2 3 3 4 4 5 5 0 0] )
      | color('green');
      | %text(1,0,'MCC','horizontalAlignment','right','verticalAlignment','bottom');
  RCChk_0_15 : Subsystem  RTWFcnName=RCChk_0_15  RTWFileName=JaevRI_Mdl_Lib  mask(RollingCounterErr){}
      mask help:
      | This block is used to check whther the input signal changes gradually from 0 to 15:
      | Input: 0~3, uint8;
      | RCErr: Rolling counter error;
      | For example,
      | input signal is 0→1→2→3→4→5→6→7→8→9→10→11→12→13→14→15→1/2/3/4/5/6/7/8/9/10/11/12/13/14/15, RCErr = 1;
      | input signal is 0→1→2→3→4→5→6→7→8→9→10→11→12→13→14→15→1→2→3→4→5→6→7→8→9→10→11→12→13→14→15→0, RCErr = 0;
      |
      | Simulink Custom Model Library, created by MCC.
      settings: AttributesFormatString=RCChk_0_15  RTWFcnNameOpts=User specified  RTWFileNameOpts=User specified
      mask Display:
      | color('blue')
      | % dpoly(1,[1 0],'z')
      | disp('\fontsize{12}0~15', 'texmode', 'on')
      | color('green');
      | text(1,0,'ITK','horizontalAlignment','right','verticalAlignment','bottom');
      | %text(1,0,'SEN','horizontalAlignment','right','verticalAlignment','bottom');
  RCChk_0_3 : Subsystem  RTWFcnName=RCChk_0_3  RTWFileName=JaevRI_Mdl_Lib  mask(RollingCounterErr){}
      mask help:
      | This block is used to check whther the input signal changes gradually from 0 to 3:
      | Input: 0~3, uint8;
      | RCErr: Rolling counter error;
      | For example, input signal is 0→1→2→3→1/2/3, RCErr = 1;
      |                     input signal is 0→1→2→3→1→2→3→0, RCErr = 0;
      |
      | Simulink Custom Model Library, created by MCC.
      settings: AttributesFormatString=RCChk_0_3  RTWFcnNameOpts=User specified  RTWFileNameOpts=User specified
      mask Display:
      | color('blue')
      | % dpoly(1,[1 0],'z')
      | disp('\fontsize{12}0~3', 'texmode', 'on')
      | color('green');
      | text(1,0,'ITK','horizontalAlignment','right','verticalAlignment','bottom');
      | %text(1,0,'SEN','horizontalAlignment','right','verticalAlignment','bottom');
  RollgCntrChk : Subsystem  RTWFcnName=RCChk_0_15  RTWFileName=JaevRI_Mdl_Lib  mask(RollgCntrChk){}
      mask help:
      | This block is used to check whther the input signal changes gradually from 0 to RollgCntrMax:
      | Input:
      | RollgCntr: Rolling counter value, uint8 data type, 0~3 or 0~15;
      | RollgCntrMax: the maximum value of rolling counter, uint8 data type, 3 or 15;
      | RollgCntrErrThd: the threshold to change the RCErr to be true;
      | Output:
      | RollgCntrErr: Rolling counter error flag;
      | For example, the RCErr will be true when any of the following conditions are met:
      | 1、RollgCntr > RollgCntrMax;
      | 2、RollgCntr maintain RollgCntrErrThd+1 steps without increasing；
      |
      | Simulink Custom Model Library, created by MCC.
      settings: AttributesFormatString=RollgCntrChk  RTWFcnNameOpts=User specified  RTWFileNameOpts=User specified
      mask Display:
      | color('blue')
      | % dpoly(1,[1 0],'z')
      | text(0.3,0.7, '0~RollgCntrMax');
      | % disp('\fontsize{10}0~RollgCntrMax', 'texmode', 'on')
      | color('green');
      | text(1,0,'ITK','horizontalAlignment','right','verticalAlignment','bottom');
      | %text(1,0,'SEN','horizontalAlignment','right','verticalAlignment','bottom');
